simulink model "PID_auto"  (R2020b)
settings: Solver=VariableStepAuto  StartTime=0.0  StopTime=30  RelTol=1e-3
values from neighbouring files (symbols this model uses):
  Fi = 1/Ti    (= 0.406504065041)    [PID_auto_script.m]    (also in autotune_PID.m = 1/Ti)
  Kp = 0.6*K_crit    (= 1.266)    [PID_auto_script.m]    (also in autotune_PID.m = 0.6*K_crit; script_PID_auto.m = 1.26)
  M = 5    [PID_auto_script.m]    (also in script_PID_auto.m)
  R = 1    [PID_auto_script.m]
  Td = T_estr/8    (= 0.615)    [PID_auto_script.m]    (also in autotune_PID.m = T_crit/8; script_PID_auto.m = 0.6125)
undefined symbols (not defined in the file or in its folder): Kp_a
libraries: cstblocks x3, pid_lib x2
settings Model: Creator=lucas  LastModifiedBy=lucas

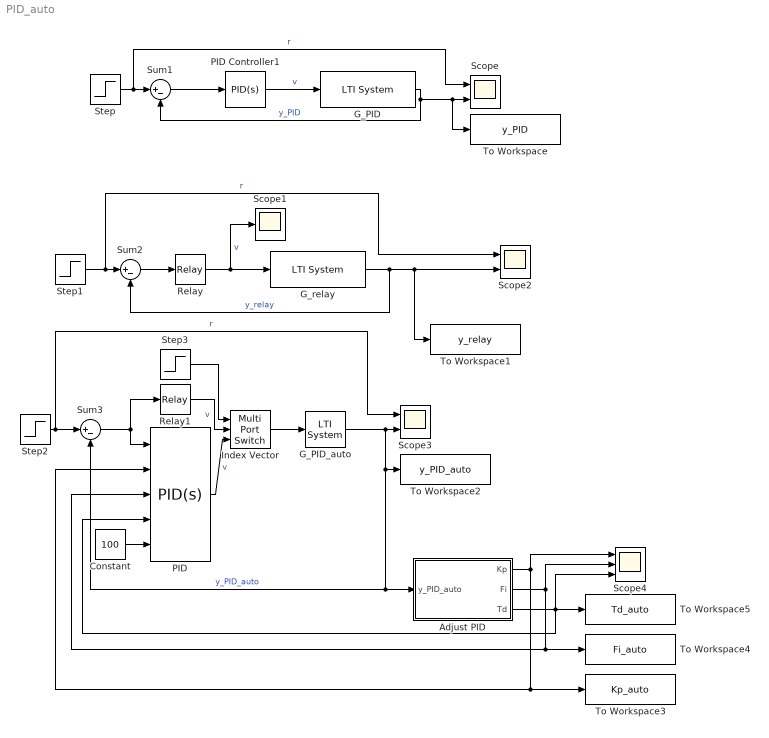
== system PID_auto ==
  Adjust PID : Subsystem
  Constant : Constant  Value=100
  G_PID : cstblocks/LTI System  sys=G  IC=[]
  G_PID_auto : cstblocks/LTI System  sys=G  IC=[]
  G_relay : cstblocks/LTI System  sys=G  IC=[]
  Index Vector : MultiPortSwitch  DataPortOrder=Zero-based contiguous  Inputs=2  zeroidx=on
  PID : pid_lib/PID Controller  Controller=PID  Form=Parallel  TimeDomain=Continuous-time  UseExternalTs=off  SampleTime=-1  IntegratorMethod=Forward Euler  FilterMethod=Forward Euler  ControllerParametersSource=external  P=Kp_a  UseFilter=on  N=100  TunerSelectOption=Transfer Function Based (PID Tuner App)  InitialConditionSource=internal  InitialConditionForIntegrator=0  InitialConditionForFilter=0  DifferentiatorICPrevScaledInput=0  ExternalReset=none  TrackingMode=off  Kt=1  LimitOutput=off  SatLimitsSource=internal  UpperSaturationLimit=inf  LowerSaturationLimit=-inf  LinearizeAsGain=on  AntiWindupMode=none  Kb=1  POutMin=[]  POutMax=[]  IOutMin=[]  IOutMax=[]  DOutMin=[]  DOutMax=[]  NOutMin=[]  NOutMax=[]  SumOutMin=[]  SumOutMax=[]  SaturationOutMin=[]  SaturationOutMax=[]  PParamMin=[]  PParamMax=[]  IParamMin=[]  IParamMax=[]  DParamMin=[]  DParamMax=[]  NParamMin=[]  NParamMax=[]  KbParamMin=[]  KbParamMax=[]  KtParamMin=[]  KtParamMax=[]  KbOutMin=[]  KbOutMax=[]  KtOutMin=[]  KtOutMax=[]  IntegratorOutMin=[]  IntegratorOutMax=[]  FilterOutMin=[]  FilterOutMax=[]  SumI1OutMin=[]  SumI1OutMax=[]  SumI2OutMin=[]  SumI2OutMax=[]  SumI3OutMin=[]  SumI3OutMax=[]  SumI4OutMin=[]  SumI4OutMax=[]  SumDOutMin=[]  SumDOutMax=[]  DifferentiatorOutMin=[]  DifferentiatorOutMax=[]  FilterDiffOutCoefMin=[]  FilterDiffOutCoefMax=[]  ReciprocalOutMin=[]  ReciprocalOutMax=[]  SumDenOutMin=[]  SumDenOutMax=[]  SumNumOutMin=[]  SumNumOutMax=[]  DivideOutMin=[]  DivideOutMax=[]  UdiffTsProdOutMin=[]  UdiffTsProdOutMax=[]  NTsProdOutMin=[]  NTsProdOutMax=[]  UintegralTsProdOutMin=[]  UintegralTsProdOutMax=[]  UngainTsProdOutMin=[]  UngainTsProdOutMax=[]  IntegratorContinuousStateAttributes=''  IntegratorStateMustResolveToSignalObject=off  IntegratorRTWStateStorageClass=Auto  FilterContinuousStateAttributes=''  FilterStateMustResolveToSignalObject=off  FilterRTWStateStorageClass=Auto  ParallelPVariant=ExternalParameters  IdealPVariant=Disabled  IVariant=ExternalParameters  DVariant=ExternalParameters  IntegratorVariant=Continuous  SatVariant=Disabled  AWVariant=Passthrough  PCopyVariant=Disabled  TRVariant=Disabled  FdbkBlocksVariant=Forward  IdealPFdbkVariant=Disabled  SatFdbkVariant=Disabled  DerivativeFilterVariant=ContFilter  NVariant=ExternalParameters  NCopyVariant=Disabled  FilterICVariant=InternalICsFilter  IntegratorICVariant=InternalICs  ExternalResetVariant=Disabled  TRSumVariant=Passthrough  SumFdbkVariant=Disabled  SumVariant=Sum_PID  TsampFilterVariant=InternalTs  TsampNgainVariant=Passthrough  TsampIntegralVariant=Passthrough  ExternalSaturationOutDataTypeStr=Inherit: Same as second input
  PID Controller1 : pid_lib/PID Controller  Controller=PID  Form=Parallel  TimeDomain=Continuous-time  UseExternalTs=off  SampleTime=-1  IntegratorMethod=Forward Euler  FilterMethod=Forward Euler  ControllerParametersSource=internal  P=Kp  I=Fi  D=Td  UseFilter=on  N=100  TunerSelectOption=Transfer Function Based (PID Tuner App)  InitialConditionSource=internal  InitialConditionForIntegrator=0  InitialConditionForFilter=0  DifferentiatorICPrevScaledInput=0  ExternalReset=none  TrackingMode=off  Kt=1  LimitOutput=off  SatLimitsSource=internal  UpperSaturationLimit=inf  LowerSaturationLimit=-inf  LinearizeAsGain=on  AntiWindupMode=none  Kb=1  POutMin=[]  POutMax=[]  IOutMin=[]  IOutMax=[]  DOutMin=[]  DOutMax=[]  NOutMin=[]  NOutMax=[]  SumOutMin=[]  SumOutMax=[]  SaturationOutMin=[]  SaturationOutMax=[]  PParamMin=[]  PParamMax=[]  IParamMin=[]  IParamMax=[]  DParamMin=[]  DParamMax=[]  NParamMin=[]  NParamMax=[]  KbParamMin=[]  KbParamMax=[]  KtParamMin=[]  KtParamMax=[]  KbOutMin=[]  KbOutMax=[]  KtOutMin=[]  KtOutMax=[]  IntegratorOutMin=[]  IntegratorOutMax=[]  FilterOutMin=[]  FilterOutMax=[]  SumI1OutMin=[]  SumI1OutMax=[]  SumI2OutMin=[]  SumI2OutMax=[]  SumI3OutMin=[]  SumI3OutMax=[]  SumI4OutMin=[]  SumI4OutMax=[]  SumDOutMin=[]  SumDOutMax=[]  DifferentiatorOutMin=[]  DifferentiatorOutMax=[]  FilterDiffOutCoefMin=[]  FilterDiffOutCoefMax=[]  ReciprocalOutMin=[]  ReciprocalOutMax=[]  SumDenOutMin=[]  SumDenOutMax=[]  SumNumOutMin=[]  SumNumOutMax=[]  DivideOutMin=[]  DivideOutMax=[]  UdiffTsProdOutMin=[]  UdiffTsProdOutMax=[]  NTsProdOutMin=[]  NTsProdOutMax=[]  UintegralTsProdOutMin=[]  UintegralTsProdOutMax=[]  UngainTsProdOutMin=[]  UngainTsProdOutMax=[]  IntegratorContinuousStateAttributes=''  IntegratorStateMustResolveToSignalObject=off  IntegratorRTWStateStorageClass=Auto  FilterContinuousStateAttributes=''  FilterStateMustResolveToSignalObject=off  FilterRTWStateStorageClass=Auto  ParallelPVariant=InternalParameters  IdealPVariant=Disabled  IVariant=InternalParameters  DVariant=InternalParameters  IntegratorVariant=Continuous  SatVariant=Disabled  AWVariant=Passthrough  PCopyVariant=Disabled  TRVariant=Disabled  FdbkBlocksVariant=Forward  IdealPFdbkVariant=Disabled  SatFdbkVariant=Disabled  DerivativeFilterVariant=ContFilter  NVariant=InternalParameters  NCopyVariant=Disabled  FilterICVariant=InternalICsFilter  IntegratorICVariant=InternalICs  ExternalResetVariant=Disabled  TRSumVariant=Passthrough  SumFdbkVariant=Disabled  SumVariant=Sum_PID  TsampFilterVariant=InternalTs  TsampNgainVariant=Passthrough  TsampIntegralVariant=Passthrough  ExternalSaturationOutDataTypeStr=Inherit: Same as second input
  Relay : Relay  OnSwitchValue=0  OffSwitchValue=0  OnOutputValue=M  OffOutputValue=-M
  Relay1 : Relay  OnSwitchValue=0  OffSwitchValue=0  OnOutputValue=M  OffOutputValue=-M
  Scope : Scope  NumInputPorts=2
  Scope1 : Scope
  Scope2 : Scope  NumInputPorts=2
  Scope3 : Scope  NumInputPorts=2
  Scope4 : Scope  NumInputPorts=3
  Step : Step  Time=0  After=R  SampleTime=0
  Step1 : Step  Time=0  After=R  SampleTime=0
  Step2 : Step  Time=0  After=R  SampleTime=0
  Step3 : Step  Time=8  SampleTime=0
  Sum1 : Sum  Inputs=|+-
  Sum2 : Sum  Inputs=|+-
  Sum3 : Sum  Inputs=|+-
  To Workspace : ToWorkspace  VariableName=y_PID  SaveFormat=Timeseries  SampleTime=-1
  To Workspace1 : ToWorkspace  VariableName=y_relay  SaveFormat=Timeseries  SampleTime=-1
  To Workspace2 : ToWorkspace  VariableName=y_PID_auto  SaveFormat=Timeseries  SampleTime=-1
  To Workspace3 : ToWorkspace  VariableName=Kp_auto  SampleTime=-1
      settings: MaxDataPoints=1  Save2DSignal=2-D array (concatenate along first dimension)
  To Workspace4 : ToWorkspace  VariableName=Fi_auto  SampleTime=-1
      settings: MaxDataPoints=1  Save2DSignal=2-D array (concatenate along first dimension)
  To Workspace5 : ToWorkspace  VariableName=Td_auto  SampleTime=-1
      settings: MaxDataPoints=1  Save2DSignal=2-D array (concatenate along first dimension)
  wires:
  Sum1/1 -> PID Controller1/1
  PID Controller1/1 -> G_PID/1  "v"
  G_PID/1 -> To Workspace/1, Scope/2, Sum1/2  "y_PID"
  Step/1 -> Scope/1, Sum1/1  "r"
  G_relay/1 -> Sum2/2, To Workspace1/1, Scope2/2  "y_relay"
  Sum2/1 -> Relay/1
  Relay/1 -> Scope1/1, G_relay/1  "v"
  Step1/1 -> Scope2/1, Sum2/1  "r"
  Sum3/1 -> PID/1, Relay1/1
  G_PID_auto/1 -> Sum3/2, Adjust PID/1(y_PID_auto), To Workspace2/1, Scope3/2  "y_PID_auto"
  Step2/1 -> Scope3/1, Sum3/1  "r"
  Relay1/1 -> Index Vector/2  "v"
  Step3/1 -> Index Vector/1
  Index Vector/1 -> G_PID_auto/1
  Adjust PID/1(Kp) -> PID/2, To Workspace3/1, Scope4/1
  Adjust PID/2(Fi) -> PID/3, To Workspace4/1, Scope4/2
  Adjust PID/3(Td) -> Scope4/3, PID/4, To Workspace5/1
  PID/1 -> Index Vector/3  "v"
  Constant/1 -> PID/5

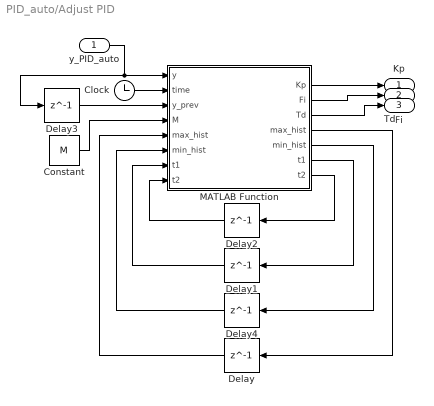
== system PID_auto/Adjust PID ==
  y_PID_auto : Inport
  Clock : Clock
  Constant : Constant  Value=M
  Delay : Delay  DelayLength=1  InitialCondition=1
  Delay1 : Delay  DelayLength=1  InitialCondition=0
  Delay2 : Delay  DelayLength=1  InitialCondition=1
  Delay3 : Delay  DelayLength=1  InitialCondition=0
  Delay4 : Delay  DelayLength=1  InitialCondition=-1
  MATLAB Function : MATLAB Function  TreatAsAtomicUnit=on
  Kp : Outport
  Fi : Outport  Port=2
  Td : Outport  Port=3
  wires:
  Delay1/1 -> MATLAB Function/7("t1 ")
  MATLAB Function/7(t2) -> Delay2/1
  Constant/1 -> MATLAB Function/4(M)
  MATLAB Function/6(t1) -> Delay1/1
  Delay3/1 -> MATLAB Function/3(y_prev)
  Clock/1 -> MATLAB Function/2(time)
  MATLAB Function/5(min_hist) -> Delay4/1
  y_PID_auto/1 -> Delay3/1, MATLAB Function/1(y)
  MATLAB Function/4(max_hist) -> Delay/1
  Delay2/1 -> MATLAB Function/8("t2 ")
  MATLAB Function/3(Td) -> Td/1
  Delay/1 -> MATLAB Function/5("max_hist ")
  Delay4/1 -> MATLAB Function/6("min_hist ")
  MATLAB Function/2(Fi) -> Fi/1
  MATLAB Function/1(Kp) -> Kp/1

== matlab function PID_auto/Adjust PID/MATLAB Function ==
  data: y input; time input; y_prev input; M input; Kp output; Fi output; Td output; max_hist input; min_hist input; max_hist output; min_hist output; t1 output; t2 output; t1 input; t2 input
function [Kp,Fi,Td,max_hist,min_hist,t1,t2] = set_PID(y,time,y_prev,M,max_hist,min_hist,t1,t2)

    if y >= max_hist
        max_hist = y;
    end
    if y <= min_hist
        min_hist = y;
    end
    if y_prev >= max_hist && y <= y_prev && time < 8
        t1 = time-1;
    end
    if y_prev <= min_hist && y >= y_prev && time < 8
        t2 = time-1;
    end
    T_crit = 2*(t2-t1);
    A_crit = (max_hist-min_hist)/2;
    K_crit = 4*M/(pi*A_crit);
    Kp = 0.6*K_crit;
    Ti = T_crit/2;
    Fi = 1/Ti;
    Td = T_crit/8;
end
